simulink model "controlador"  (Simulink 7.9)
settings: Solver=ode45  StartTime=0.0  StopTime=150  RelTol=1e-3
settings Model: Creator=Miguel Faggioni  LastModifiedBy=Miguel Faggioni
settings DataIOCC: TimeSaveName=t

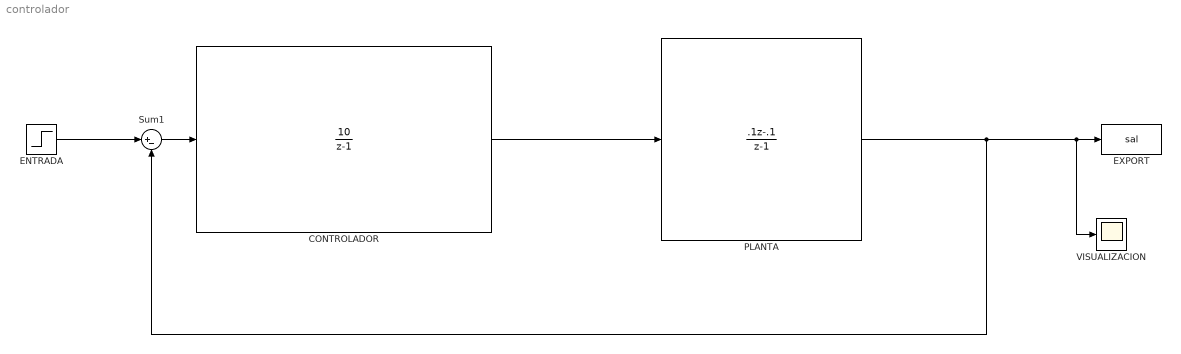
== system controlador ==
  CONTROLADOR : DiscreteTransferFcn  Numerator=[10]  Denominator="[1  -1]"
  ENTRADA : Step  Time=0  After=5  SampleTime=.5
  EXPORT : ToWorkspace  VariableName=sal  SampleTime=-1
  PLANTA : DiscreteTransferFcn  Numerator=[.1 -.1]  Denominator=[1 -1]
  Sum1 : Sum  Inputs=|+-
  VISUALIZACION : Scope
      settings: TimeRange=10  YMin=-4e+38  YMax=0
  wires:
  ENTRADA/1 -> Sum1/1
  Sum1/1 -> CONTROLADOR/1
  PLANTA/1 -> Sum1/2, EXPORT/1, VISUALIZACION/1
  CONTROLADOR/1 -> PLANTA/1
